simulink model "power_paralbranch"  (Simulink 6.0)
settings: Solver=ode23s  SolverMode=SingleTasking  StartTime=0.0  StopTime=0.1  RelTol=1e-3  AbsTol=1e-6
libraries: powerlib x7
settings Model: Creator=patrice  LastModifiedBy=batserve  ExtModeTrigMode=oneshot  ExtModeArmWhenConnect=off  ExtModeAutoUpdateStatusClock=off
settings DataIOCC: LimitDataPoints=off  SignalLoggingName=sigsOut
settings OptimizationCC: BooleanDataType=off
settings DebuggingCC: SolverPrmCheckMsg=none
settings HardwareCC: TargetUnknown=on
settings RTWCC: TemplateMakefile=grt_unix.tmf

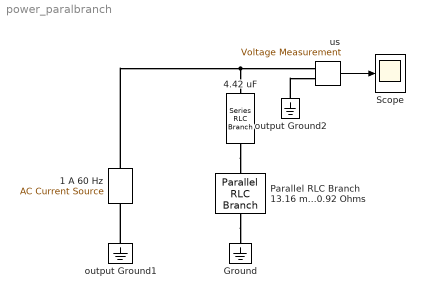
== system power_paralbranch ==
  1 A 60 Hz : powerlib/Electrical Sources/AC Current Source  Orientation=up  Amplitude=1  Phase=0  Frequency=60  SampleTime=0  Measurements=None
      settings: AttributesFormatString=\n
  4.42 uF : powerlib/Elements/Series RLC Branch  Orientation=down  PhysicalDomain=powersysdomain  SubClassName=unknown  PortType=p1  LConnTagsString=__new0  RConnTagsString=__new0  Resistance=0  Inductance=0  Capacitance=4.42e-06  Measurements=None
  Ground : powerlib/Elements/Ground  Orientation=down  PhysicalDomain=powersysdomain  SubClassName=unknown  PortType=p1  LConnTagsString=a
  Parallel RLC Branch 13.16 mH  70.92 Ohms : powerlib/Elements/Parallel RLC Branch  Orientation=down  PhysicalDomain=powersysdomain  SubClassName=unknown  PortType=p1  LConnTagsString=a  RConnTagsString=__new0  Resistance=70.92  Inductance=13.16e-03  Capacitance=0  Measurements=None
  Scope : Scope
      settings: TickLabels=on  TimeRange=0.1  YMin=-1000  YMax=1000  DataFormat=Array
  output Ground1 : powerlib/Elements/Ground  Orientation=down  PhysicalDomain=powersysdomain  SubClassName=unknown  PortType=p1  LConnTagsString=a
  output Ground2 : powerlib/Elements/Ground  Orientation=down  PhysicalDomain=powersysdomain  SubClassName=unknown  PortType=p1  LConnTagsString=a
  us : powerlib/Measurements/Voltage Measurement  Tag=PoWeRsYsTeMmEaSuReMeNt  PhasorSimulation=off  OutputType=Magnitude  PSBequivalent=0
  wires:
  us/1 -> Scope/1
  connections:
  1 A 60 Hz/RConn1 -- 4.42 uF/LConn1 -- us/LConn1
  4.42 uF/RConn1 -- Parallel RLC Branch 13.16 mH  70.92 Ohms/LConn1
  Parallel RLC Branch 13.16 mH  70.92 Ohms/RConn1 -- Ground/LConn1
  output Ground1/LConn1 -- 1 A 60 Hz/LConn1
  output Ground2/LConn1 -- us/LConn2
